simulink library "HY_General_Library"  (R2018b)
settings: Solver=ode45  StartTime=0.0  StopTime=10.0  RelTol=1e-3  EnableMultiTasking=on
undefined symbols (not defined in the file or in its folder): dT, Slope1, Slope2
libraries: simulink x63, $bdroot x4
(part 5 of 5)

== system HY_General_Library/Debounce_Blocks/Debounce_OBD_FCN_St/Debounce_OBD/counterRst ==
  note: rising edge detection
  note: only if the FaultDetectionCounter less than 0
  note: test run failure always causes fault detection counter to increment above 0
      | (so as not to double the fail detection time following a test complete with pass)
  bErr : Inport
  z_1 : Inport  Port=2
  ConstOne1 : Constant  Description=TOPexpert TAT block library for modelling of ECU functions - (c) by FEV - all rights reserved. Confidential - no passing on third parties, Calibration Methods (TEM), 2003-2006, schoenfelder  InitFcn=try;p = get_param(gcb,'Ports'); p = p(1);posblk = get_param(gcb,'Position');set_param(gcb,'Position',[posblk(1) posblk(2) posblk(1)+25 posblk(2)+15]);end;  Value=0  OutDataTypeStr=int16
      settings: AttributesFormatString=%<OutDataTypeStr>
  ConstOne10 : Constant  Description=TOPexpert TAT block library for modelling of ECU functions - (c) by FEV - all rights reserved. Confidential - no passing on third parties, Calibration Methods (TEM), 2003-2006, schoenfelder  InitFcn=try;p = get_param(gcb,'Ports'); p = p(1);posblk = get_param(gcb,'Position');set_param(gcb,'Position',[posblk(1) posblk(2) posblk(1)+25 posblk(2)+15]);end;  Value=0  OutDataTypeStr=int16
      settings: AttributesFormatString=%<OutDataTypeStr>
  Logical Operator : Logic  AllPortsSameDT=off  OutDataTypeStr=boolean
  Relational Operator : RelationalOperator  Operator=<  OutDataTypeStr=boolean  RndMeth=Nearest
  Relational Operator1 : RelationalOperator  Operator=>  OutDataTypeStr=boolean  RndMeth=Nearest
  SwCtrResetDurFail : Switch  Criteria=u2 ~= 0  SaturateOnIntegerOverflow=on  InputSameDT=on
      settings: AttributesFormatString=%<Criteria>
  Unit Delay1 : UnitDelay  SampleTime=-1
      settings: AttributesFormatString=Init: %<X0>
  Out : Outport
  wires:
  z_1/1 -> Relational Operator/1, SwCtrResetDurFail/3
  ConstOne1/1 -> SwCtrResetDurFail/1
  Unit Delay1/1 -> Relational Operator1/2
  Relational Operator1/1 -> Logical Operator/1
  ConstOne10/1 -> Relational Operator/2
  Relational Operator/1 -> Logical Operator/2
  Logical Operator/1 -> SwCtrResetDurFail/2
  bErr/1 -> Relational Operator1/1, Unit Delay1/1
  SwCtrResetDurFail/1 -> Out/1

== system HY_General_Library/Debounce_Blocks/Debounce_OBD_FCN_St/Debounce_OBD/errorLevel ==
  bTestNotCompleted : Inport
  bFailed : Inport  Port=2
  bErrCfm : Inport  Port=3
  bWarnIndAcv : Inport  Port=4
  Constant1 : Constant  OutDataTypeStr=uint8
      settings: AttributesFormatString=%<OutDataTypeStr>
  Constant{2,4,6,8} (4 alike) : Constant  Value=0  OutDataTypeStr=uint8
      settings: AttributesFormatString=%<OutDataTypeStr>
  Constant3 : Constant  Value=10  OutDataTypeStr=uint8
      settings: AttributesFormatString=%<OutDataTypeStr>
  Constant5 : Constant  Value=128  OutDataTypeStr=uint8
      settings: AttributesFormatString=%<OutDataTypeStr>
  Constant7 : Constant  Value=64  OutDataTypeStr=uint8
      settings: AttributesFormatString=%<OutDataTypeStr>
  Logical Operator : Logic  AllPortsSameDT=off  OutDataTypeStr=boolean
  Sum1 : Sum  Inputs=++++  AccumDataTypeStr=uint8  OutDataTypeStr=uint8  SaturateOnIntegerOverflow=on
  Switch{1,3..5} (4 alike) : Switch  Criteria=u2 ~= 0  SaturateOnIntegerOverflow=on  InputSameDT=on
      settings: AttributesFormatString=%<Criteria>
  stDgo : Outport
  wires:
  bTestNotCompleted/1 -> Switch1/2
  bWarnIndAcv/1 -> Logical Operator/2
  bFailed/1 -> Logical Operator/1, Switch3/2
  Constant1/1 -> Switch3/1
  Constant2/1 -> Switch3/3
  bErrCfm/1 -> Switch4/2
  Constant3/1 -> Switch4/1
  Constant4/1 -> Switch4/3
  Switch3/1 -> Sum1/1
  Switch4/1 -> Sum1/2
  Sum1/1 -> stDgo/1
  Constant5/1 -> Switch5/1
  Constant6/1 -> Switch5/3
  Switch5/1 -> Sum1/3
  Logical Operator/1 -> Switch5/2
  Constant7/1 -> Switch1/1
  Constant8/1 -> Switch1/3
  Switch1/1 -> Sum1/4

== system HY_General_Library/PID_Blocks/PositionPID/Subsystem1/Subsystem ==
  Err : Inport
  PreSat : Inport  Port=2
  UpperSatLimd : Inport  Port=3
  LowerSatLimd : Inport  Port=4
  CtrlIntgVal : Inport  Port=5
  AND : Logic  DisableCoverage=on  OutDataTypeStr=boolean
  AND1 : Logic  DisableCoverage=on  Operator=OR  OutDataTypeStr=boolean
  Constant1 : Constant  Value=0  OutDataTypeStr=single
  DataTypeConv3 : DataTypeConversion  DisableCoverage=on  OutDataTypeStr=int8
  DataTypeConv4 : DataTypeConversion  DisableCoverage=on  OutDataTypeStr=int8
  Multiport Switch1 : MultiPortSwitch  DataPortOrder=Zero-based contiguous  Inputs=2  zeroidx=on
  Product2 : Product
  Relational Operator1 : RelationalOperator  Operator=>  OutDataTypeStr=boolean  RndMeth=Nearest
  Relational Operator2 : RelationalOperator  Operator===  OutDataTypeStr=boolean  RndMeth=Simplest
  Relational Operator3 : RelationalOperator  Operator=<  OutDataTypeStr=boolean  RndMeth=Nearest
  SignPreIntegrator1 : Signum  DisableCoverage=on
  SignPreIntegrator2 : Signum  DisableCoverage=on
  Out : Outport
  wires:
  AND1/1 -> AND/1
  Constant1/1 -> Multiport Switch1/3
  Multiport Switch1/1 -> Out/1
  Err/1 -> Product2/1, SignPreIntegrator2/1
  AND/1 -> Multiport Switch1/1
  Relational Operator2/1 -> AND/2
  SignPreIntegrator1/1 -> DataTypeConv3/1
  DataTypeConv3/1 -> Relational Operator2/1
  DataTypeConv4/1 -> Relational Operator2/2
  SignPreIntegrator2/1 -> DataTypeConv4/1
  PreSat/1 -> Relational Operator1/1, Relational Operator3/1, SignPreIntegrator1/1
  LowerSatLimd/1 -> Relational Operator3/2
  Relational Operator1/1 -> AND1/1
  UpperSatLimd/1 -> Relational Operator1/2
  Relational Operator3/1 -> AND1/2
  Product2/1 -> Multiport Switch1/2
  CtrlIntgVal/1 -> Product2/2

== system HY_General_Library/Debounce_Blocks/Debounce_OBD_FCN/Debounce_OBD/Relay/SRFlipFlop ==
  S : Inport
  R : Inport  Port=2
  SRNOR : Logic  Operator=NOR  AllPortsSameDT=off  OutDataTypeStr=boolean
  SRNOR1 : Logic  Operator=NOR  AllPortsSameDT=off  OutDataTypeStr=boolean
  Unit Delay : UnitDelay  SampleTime=-1
      settings: AttributesFormatString=<initial=%<X0>>
  Q : Outport
  wires:
  SRNOR1/1 -> Unit Delay/1, Q/1
  S/1 -> SRNOR/1
  SRNOR/1 -> SRNOR1/2
  Unit Delay/1 -> SRNOR/2
  R/1 -> SRNOR1/1

== system HY_General_Library/Debounce_Blocks/Debounce_OBD_FCN_St/Debounce_OBD/Relay/SRFlipFlop ==
  S : Inport
  R : Inport  Port=2
  SRNOR : Logic  Operator=NOR  AllPortsSameDT=off  OutDataTypeStr=boolean
  SRNOR1 : Logic  AllPortsSameDT=off  OutDataTypeStr=boolean
  SRNOR2 : Logic  Operator=NOT  Inputs=1  AllPortsSameDT=off  OutDataTypeStr=boolean
  Unit Delay : UnitDelay  SampleTime=-1
      settings: AttributesFormatString=Init: %<X0>
  Q : Outport
  wires:
  R/1 -> SRNOR2/1
  SRNOR1/1 -> Unit Delay/1, Q/1
  S/1 -> SRNOR/1
  SRNOR/1 -> SRNOR1/2
  Unit Delay/1 -> SRNOR/2
  SRNOR2/1 -> SRNOR1/1

== system HY_General_Library/Debounce_Blocks/Debounce_OBD_FCN_St/Debounce_OBD/Relay/SRFlipFlop1 ==
  S : Inport
  R : Inport  Port=2
  SRNOR : Logic  Operator=NOR  AllPortsSameDT=off  OutDataTypeStr=boolean
  SRNOR1 : Logic  AllPortsSameDT=off  OutDataTypeStr=boolean
  SRNOR2 : Logic  Operator=NOT  Inputs=1  AllPortsSameDT=off  OutDataTypeStr=boolean
  Unit Delay : UnitDelay  SampleTime=-1
      settings: AttributesFormatString=Init: %<X0>
  Q : Outport
  wires:
  SRNOR2/1 -> SRNOR1/1
  Unit Delay/1 -> SRNOR/2
  SRNOR/1 -> SRNOR1/2
  S/1 -> SRNOR/1
  SRNOR1/1 -> Q/1, Unit Delay/1
  R/1 -> SRNOR2/1
